simulink model "Systeem_Identificatie_Data_Uitlezen"  (R2018b)
settings: Solver=FixedStepAuto  StartTime=0.0  StopTime=4  FixedStep=1/100000  RelTol=1e-3
libraries: dspnetwork x1
settings Model: Creator=Roberto  LastModifiedBy=Roberto
settings DataIOCC: SaveTime=off

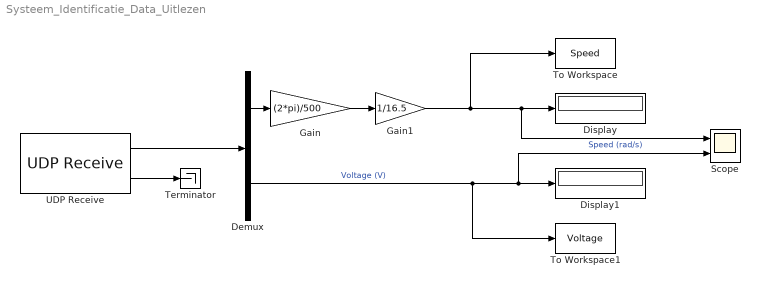
== system Systeem_Identificatie_Data_Uitlezen ==
  Demux : Demux  Outputs=2
  Display : Display
  Display1 : Display
  Gain : Gain  Gain=(2*pi)/500
  Gain1 : Gain  Gain=1/16.5
  Scope : Scope  NumInputPorts=2
  Terminator : Terminator
  To Workspace : ToWorkspace  VariableName=Speed  SampleTime=1/50000
      settings: Save2DSignal=2-D array (concatenate along first dimension)
  To Workspace1 : ToWorkspace  VariableName=Voltage  SampleTime=1/50000
      settings: Save2DSignal=2-D array (concatenate along first dimension)
  UDP Receive : dspnetwork/UDP Receive  localURL='0.0.0.0'  localPort=25002  remoteURL='0.0.0.0'  remotePort=-1  recvBufferSize=8192  dims=2  signalDatatype=double  isVarSize=off  showBlockingTime=on  blockingTime=2  sampletime=1/50000  blockPlatform=HOST
      settings: SourceProductName=DSP System Toolbox  SourceProductBaseCode=DS
  wires:
  UDP Receive/2 -> Terminator/1
  UDP Receive/1 -> Demux/1
  Demux/1 -> Gain/1
  Demux/2 -> To Workspace1/1, Scope/2, Display1/1  "Voltage (V)"
  Gain/1 -> Gain1/1
  Gain1/1 -> To Workspace/1, Display/1, Scope/1  "Speed (rad/s)"
